simulink model "proj_sim1"  (R2024b)
settings: Solver=VariableStepAuto  StartTime=0.0  StopTime=5  RelTol=1e-3
settings Model: Creator=Dheeraj  LastModifiedBy=Dheeraj

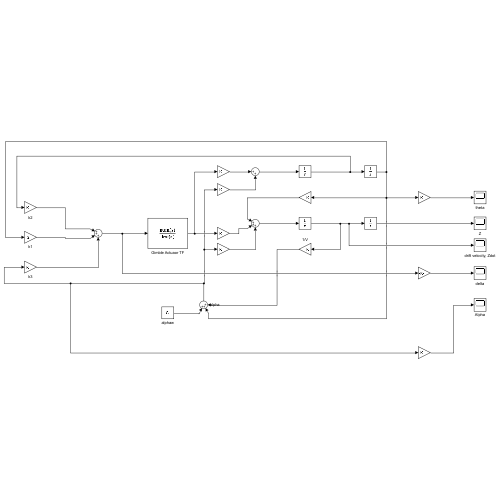
[thumbnail: Simulink's stored preview of the top-level diagram]
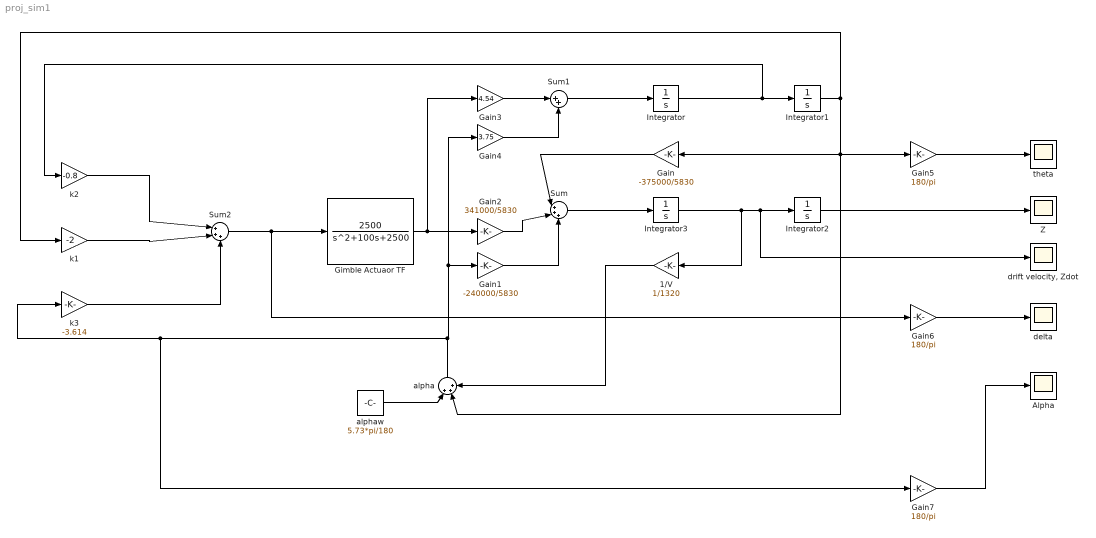
== system proj_sim1 ==
  1/V : Gain  Gain=1/1320
  Alpha : Scope
  Gain : Gain  Gain=-375000/5830
  Gain1 : Gain  Gain=-240000/5830
  Gain2 : Gain  Gain=341000/5830
  Gain3 : Gain  Gain=4.54
  Gain4 : Gain  Gain=3.75
  Gain5 : Gain  Gain=180/pi
  Gain6 : Gain  Gain=180/pi
  Gain7 : Gain  Gain=180/pi
  Gimble Actuaor TF : TransferFcn  Numerator=[2500]  Denominator=[1 100 2500]
  Integrator{,1..3} (4 alike) : Integrator
  Sum : Sum  Inputs=|+++
  Sum1 : Sum  Inputs=|++
  Sum2 : Sum  Inputs=|+++
  Z : Scope
  alpha : Sum  Inputs=|+++
  alphaw : Constant  Value=5.73*pi/180
  delta : Scope
  "drift velocity, Zdot" : Scope
  k1 : Gain  Gain=-2
  k2 : Gain  Gain=-0.8
  k3 : Gain  Gain=-3.614
  theta : Scope
  wires:
  Integrator/1 -> Integrator1/1, k2/1
  Integrator1/1 -> k1/1, alpha/2, Gain/1, Gain5/1
  Gain/1 -> Sum/1
  Sum/1 -> Integrator3/1
  alphaw/1 -> alpha/1
  1/V/1 -> alpha/3
  alpha/1 -> Gain4/1, Gain1/1, k3/1, Gain7/1
  Gain1/1 -> Sum/3
  Gain2/1 -> Sum/2
  Sum1/1 -> Integrator/1
  Gain3/1 -> Sum1/1
  Gain4/1 -> Sum1/2
  Gimble Actuaor TF/1 -> Gain3/1, Gain2/1
  Integrator2/1 -> Z/1
  Sum2/1 -> Gain6/1, Gimble Actuaor TF/1
  k1/1 -> Sum2/2
  k2/1 -> Sum2/1
  k3/1 -> Sum2/3
  Integrator3/1 -> 1/V/1, "drift velocity, Zdot"/1, Integrator2/1
  Gain5/1 -> theta/1
  Gain6/1 -> delta/1
  Gain7/1 -> Alpha/1
